simulink library "HouseThermal_lib"  (R2019a)
settings: Solver=VariableStepAuto  StartTime=0.0  StopTime=10.0  RelTol=1e-3
libraries: sl_kafka_lib x4, simulink x1
settings Model: Creator=asolland  LastModifiedBy=asolland

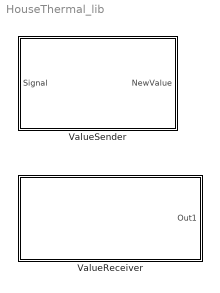
== system HouseThermal_lib ==
  ValueReceiver : Subsystem  mask{prmBroker=localhost:9092, prmTopicName=iot.forwardtemp.house}
      mask prompts: prmBroker "Kafka broker"; prmTopicName "Topic name"
      mask Display:
      | fprintf('Broker: %s\nTopic: %s', ...
      |     prmBroker, prmTopicName)
  ValueSender : Subsystem  mask{prmBroker=localhost:9092, prmTopicName=iot.forwardtemp.house, prmTopicKey=house1}
      mask prompts: prmBroker "Kafka broker"; prmTopicName "Topic name"; prmTopicKey "Topic key"
      mask Display:
      | fprintf('Broker: %s\nTopic: %s\nKey: %s', ...
      |     prmBroker, prmTopicName, prmTopicKey)

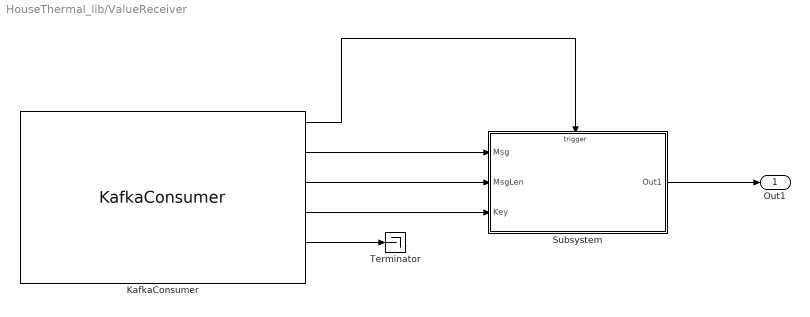
== system HouseThermal_lib/ValueReceiver ==
  KafkaConsumer : sl_kafka_lib/KafkaConsumer  sfpBrokers=prmBroker  sfpTopic=prmTopicName  sfpGroup='abc'  sfpMsgLen=128  sfpKeyLen=32  sfpOutputTimestamp=on  sfpTS=.1
      settings: SourceProductName=Kafka Library
  Subsystem : Subsystem
  Terminator : Terminator
  Out1 : Outport
  wires:
  KafkaConsumer/3 -> Subsystem/2(MsgLen)
  KafkaConsumer/5 -> Terminator/1
  KafkaConsumer/2 -> Subsystem/1(Msg)
  Subsystem/1(Out1) -> Out1/1
  KafkaConsumer/4 -> Subsystem/3(Key)
  KafkaConsumer/1 -> Subsystem/Trigger

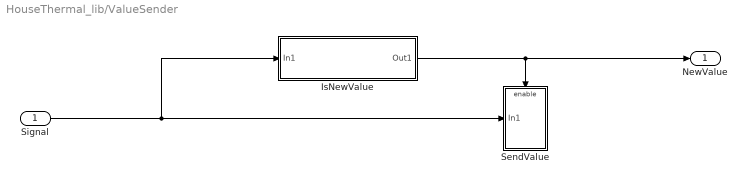
== system HouseThermal_lib/ValueSender ==
  Signal : Inport
  IsNewValue : Subsystem
  SendValue : Subsystem
  NewValue : Outport
  wires:
  Signal/1 -> SendValue/1(In1), IsNewValue/1(In1)
  IsNewValue/1(Out1) -> NewValue/1, SendValue/Enable

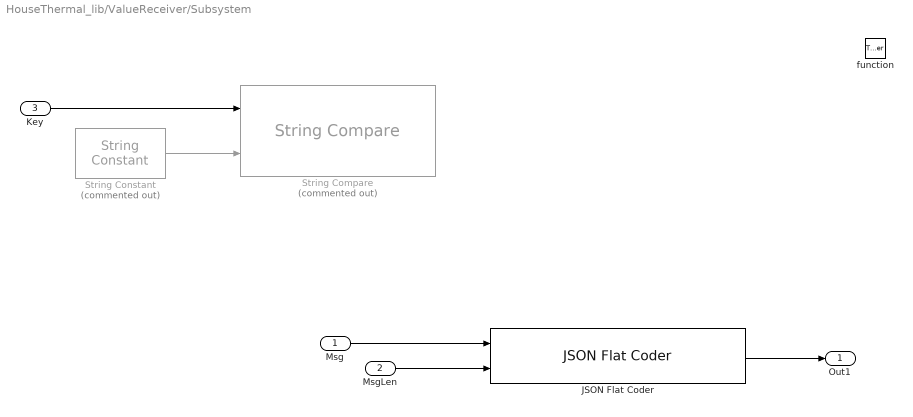
== system HouseThermal_lib/ValueReceiver/Subsystem ==
  Msg : Inport
  MsgLen : Inport  Port=2
  Key : Inport  Port=3
  function : TriggerPort  TriggerType=function-call  VariantControl=Variant
  JSON Flat Coder : sl_kafka_lib/JSON Flat Coder  sfpDirection=Decode  sfpLength=128  sfpFields={'Temp'}  sfpOutLength=on  sfpInLength=on
      settings: SourceProductName=Kafka Library
  String Compare : StringCompare  Commented=on  CompareOption=First N characters  NumberOfCharacters=6
  String Constant : StringConstant  Commented=on  String="\"house1\""
  Out1 : Outport  InitialOutput=57.1
  wires:
  Msg/1 -> JSON Flat Coder/1
  JSON Flat Coder/1 -> Out1/1
  String Constant/1 -> String Compare/2
  Key/1 -> String Compare/1
  MsgLen/1 -> JSON Flat Coder/2

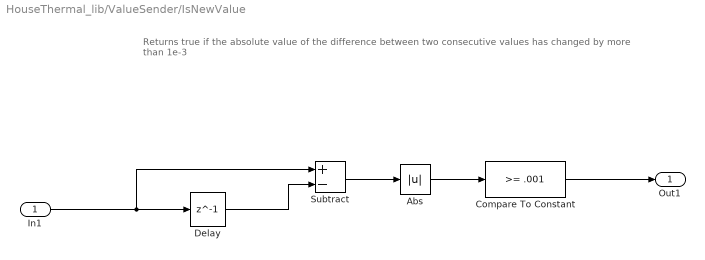
== system HouseThermal_lib/ValueSender/IsNewValue ==
  note: Returns true if the absolute value of the difference
      | between two consecutive values has changed by
      | more than 1e-3
  In1 : Inport
  Abs : Abs
  Compare To Constant : simulink/Logic and Bit Operations/Compare To Constant  relop=>=  const=.001  OutDataTypeStr=boolean
  Delay : Delay  DelayLength=1  InitialCondition=-exp(10)
  Subtract : Sum  Inputs=+-
  Out1 : Outport
  wires:
  Subtract/1 -> Abs/1
  Compare To Constant/1 -> Out1/1
  Delay/1 -> Subtract/2
  Abs/1 -> Compare To Constant/1
  In1/1 -> Delay/1, Subtract/1

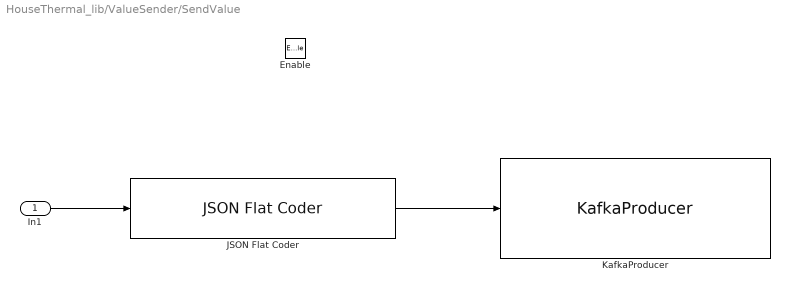
== system HouseThermal_lib/ValueSender/SendValue ==
  In1 : Inport
  Enable : EnablePort
  JSON Flat Coder : sl_kafka_lib/JSON Flat Coder  sfpDirection=Encode  sfpLength=128  sfpFields={'Temp'}  sfpOutLength=off  sfpInLength=on
      settings: SourceProductName=Kafka Library
  KafkaProducer : sl_kafka_lib/KafkaProducer  sfpBrokers=prmBroker  sfpTopic=prmTopicName  sfpKeyAsInput=off  sfpKeyAsInputLen=16  sfpKey=prmTopicKey  sfpMsgLen=128  sfpTS=-1
      settings: SourceProductName=Kafka Library
  wires:
  In1/1 -> JSON Flat Coder/1
  JSON Flat Coder/1 -> KafkaProducer/1
